simulink model "PID_Tuning_1"  (R2016a)
settings: Solver=VariableStepAuto  StartTime=0.0  StopTime=10.0  RelTol=1e-3
values from neighbouring files (symbols this model uses):
  b = 10    [Tut_Week_5.m]
  D = 0.53908    [Tut_Week_5.m]
  I = 25.0289    [Tut_Week_5.m]
  k = 20    [Tut_Week_5.m]
  M = 1    [Tut_Week_5.m]
  N = 6.4951    [Tut_Week_5.m]    (also in Week_8_Final.m = 20)
  P = 15.376    [Tut_Week_5.m]
libraries: simulink x1
settings Model: Creator=김태욱  LastModifiedBy=김태욱

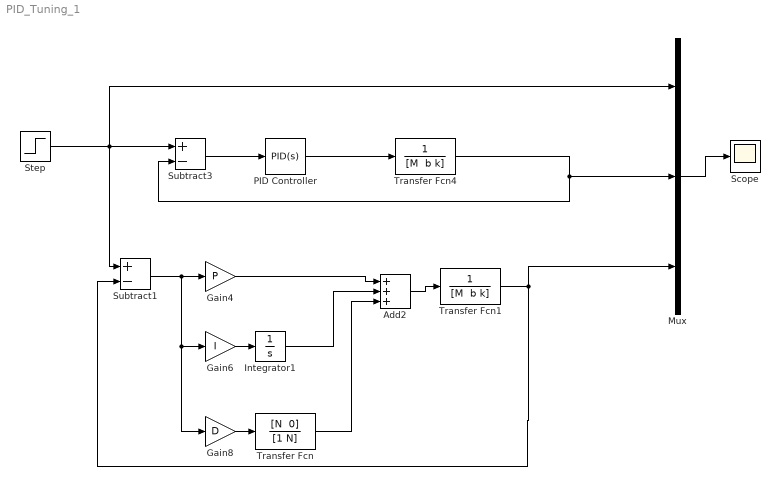
== system PID_Tuning_1 ==
  Add2 : Sum  Inputs=+++
  Gain4 : Gain  Gain=P
  Gain6 : Gain  Gain=I
  Gain8 : Gain  Gain=D
  Integrator1 : Integrator
  Mux : Mux  Inputs=3
  PID Controller : simulink/Continuous/PID Controller  Controller=PID  TimeDomain=Continuous-time  SampleTime=-1  IntegratorMethod=Forward Euler  FilterMethod=Forward Euler  Form=Parallel  UseFilter=on  ControllerParametersSource=internal  P=1  I=1  D=0  N=100  InitialConditionSource=internal  InitialConditionForIntegrator=0  InitialConditionForFilter=0  ExternalReset=none  LimitOutput=off  UpperSaturationLimit=inf  LowerSaturationLimit=-inf  LinearizeAsGain=on  AntiWindupMode=none  Kb=1  TrackingMode=off  Kt=1  PParamMin=[]  PParamMax=[]  IParamMin=[]  IParamMax=[]  DParamMin=[]  DParamMax=[]  NParamMin=[]  NParamMax=[]  KbParamMin=[]  KbParamMax=[]  KtParamMin=[]  KtParamMax=[]  POutMin=[]  POutMax=[]  IOutMin=[]  IOutMax=[]  DOutMin=[]  DOutMax=[]  NOutMin=[]  NOutMax=[]  KbOutMin=[]  KbOutMax=[]  KtOutMin=[]  KtOutMax=[]  IntegratorOutMin=[]  IntegratorOutMax=[]  FilterOutMin=[]  FilterOutMax=[]  SumOutMin=[]  SumOutMax=[]  SumI1OutMin=[]  SumI1OutMax=[]  SumI2OutMin=[]  SumI2OutMax=[]  SumI3OutMin=[]  SumI3OutMax=[]  SumDOutMin=[]  SumDOutMax=[]  SaturationOutMin=[]  SaturationOutMax=[]  IntegratorContinuousStateAttributes=''  IntegratorStateMustResolveToSignalObject=off  IntegratorRTWStateStorageClass=Auto  FilterContinuousStateAttributes=''  FilterStateMustResolveToSignalObject=off  FilterRTWStateStorageClass=Auto  DifferentiatorICPrevScaledInput=0  DifferentiatorOutMin=[]  DifferentiatorOutMax=[]
  Scope : Scope
  Step : Step  SampleTime=0
  Subtract1 : Sum  Inputs=+-
  Subtract3 : Sum  Inputs=+-
  Transfer Fcn : TransferFcn  Numerator="[N  0]"  Denominator=[1 N]
  Transfer Fcn1 : TransferFcn  Denominator="[M  b k]"
  Transfer Fcn4 : TransferFcn  Denominator="[M  b k]"
  wires:
  PID Controller/1 -> Transfer Fcn4/1
  Subtract3/1 -> PID Controller/1
  Transfer Fcn4/1 -> Subtract3/2, Mux/2
  Step/1 -> Subtract1/1, Mux/1, Subtract3/1
  Mux/1 -> Scope/1
  Gain4/1 -> Add2/1
  Add2/1 -> Transfer Fcn1/1
  Transfer Fcn1/1 -> Subtract1/2, Mux/3
  Gain6/1 -> Integrator1/1
  Integrator1/1 -> Add2/2
  Subtract1/1 -> Gain6/1, Gain8/1, Gain4/1
  Gain8/1 -> Transfer Fcn/1
  Transfer Fcn/1 -> Add2/3
